simulink model "RocketSimAA"  (R2021a)
settings: Solver=VariableStepAuto  StartTime=0.0  StopTime=100  RelTol=1e-3
values from neighbouring files (symbols this model uses):
  flag_AA = 1    [main_simulation.m]
  flag_D = 1    [main_simulation.m]
  h_lim = 1000    [main_simulation.m]
  T_s = 0.01    [main_simulation.m]
undefined symbols (not defined in the file or in its folder): A_AAbig, A_AAsmall, A_R, C_DR, Controller, f_motor, g_0, H_0, h_0, h_table, m_0, m_motor, n_finAA, phi_0, R_E, rho_0, t_BO, t_data, t_motor, theta_0, v_vec
libraries: simulink x2
settings Model: SimulationMode=accelerator  Creator=SeverinBeger  LastModifiedBy=SeverinBeger

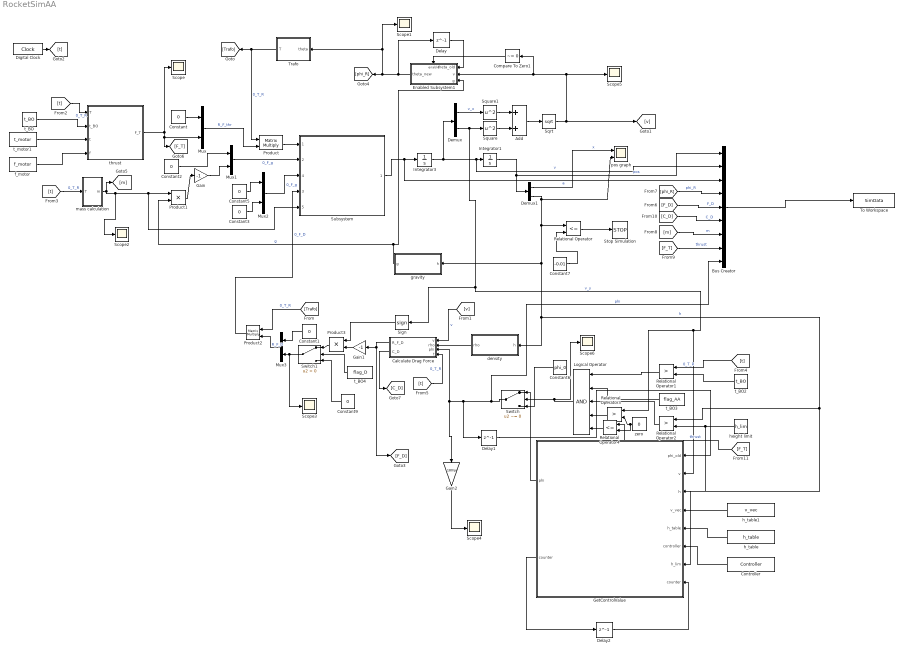
== system RocketSimAA ==
  Add : Sum
  Bus Creator : BusCreator  Inputs=9
  Calculate Drag Force : Subsystem
  Compare To Zero1 : simulink/Logic and Bit Operations/Compare To Zero  relop=~=  OutDataTypeStr=boolean
  Constant{,1..3,5,9} (6 alike) : Constant  Value=0
  Constant6 : Constant  Value=phi_0
  Constant7 : Constant  Value=-0.01
  Controller : Constant  Value=Controller
  Delay : Delay  DelayLength=1  InitialCondition=0
  Delay1 : Delay  DelayLength=1  InitialCondition=0
  Delay2 : Delay  DelayLength=1  InitialCondition=0
  Demux : Demux  Outputs=2
  Demux1 : Demux  Outputs=2
  Digital Clock : DigitalClock  SampleTime=T_s
  Enabled Subsystem1 : Subsystem  TreatAsAtomicUnit=on
  Gain : Gain  Gain=-1
  Gain1 : Gain  Gain=-1
  Gain2 : Gain  Gain=180/pi
  GetControlValue : MATLAB Function  TreatAsAtomicUnit=on
  Integrator1 : Integrator
  Integrator3 : Integrator
  Logical Operator : Logic  Inputs=5  AllPortsSameDT=off  OutDataTypeStr=boolean
  Mux{,1..3} (4 alike) : Mux  Inputs=2
  Product : Product  Multiplication=Matrix(*)
  Product1 : Product
  Product2 : Product  Multiplication=Matrix(*)
  Product3 : Product
  Relational Operator : RelationalOperator  Operator=<=  OutDataTypeStr=boolean  RndMeth=Simplest
  Relational Operator1 : RelationalOperator  Operator=>  OutDataTypeStr=boolean  RndMeth=Simplest
  Relational Operator2 : RelationalOperator  Operator=>  OutDataTypeStr=boolean  RndMeth=Simplest
  Relational Operator3 : RelationalOperator  Operator=>  OutDataTypeStr=boolean  RndMeth=Simplest
  Relational Operator4 : RelationalOperator  Operator=<=  OutDataTypeStr=boolean  RndMeth=Simplest
  Scope{,1..6} (7 alike) : Scope
  Sign : Signum
  Sqrt : Sqrt  SaturateOnIntegerOverflow=on
  Square : Math  Operator=square  SaturateOnIntegerOverflow=on
  Square1 : Math  Operator=square  SaturateOnIntegerOverflow=on
  Stop Simulation : Stop
  Subsystem : Subsystem  ReferencedSubsystem=acceleration
      settings: PortSchema="{\"entries\":[{\"content\":{\"sides\":[{\"content\":{\"connectorIds\":[\"In1\",\"In2\",\"In4\",\"In3\",\"In5\"]},\"type\":\"ConnectorPlacement.EquallySpacedRectSide\",\"uuid\":\"9ef3e48b-891b-4d0d-a708-ee121c0097dd\"},{\"content\":{\"connectorIds\":[\"Out1\"],\"side\":\"RIGHT\"},\"type\":\"ConnectorPlacement.EquallySpacedRectSide\",\"uuid\":\"fe012b3b-856e-4c20-af45-176b50db60e5\"},{\"content\":{\"connectorIds\":[],\"side\":\"TOP\"},\"type\":\"ConnectorPlacement.EquallySpacedRectSide\",\"uuid\":\"c344a42b-cb7d-481a-b552-86bd89250f10\"}]},\"type\":\"ConnectorPlacement.EquallySpacedConnector\",\"uuid\":\"b7d8efea-7233-4c8a-80e4-a1935eebb6ed\"}],\"packageUris\":[\"http://schema.mathworks.com/mf0/Connector/R2020b\"],\"version\":\"1.0\"}"
  Switch : Switch  Criteria=u2 ~= 0
  Switch1 : Switch  Criteria=u2 > Threshold
  To Workspace : ToWorkspace  VariableName=SimData  SaveFormat=Timeseries  SampleTime=-1
  Trafo : MATLAB Function  TreatAsAtomicUnit=on
  density : Subsystem
  f_motor : Constant  Value=f_motor
  gravity : Subsystem
  h_table : Constant  Value=h_table
  h_table1 : Constant  Value=v_vec
  height limit : Constant  Value=h_lim
  mass calculation : Subsystem
  pos graph : Scope  NumInputPorts=2
  t_BO : Constant  Value=t_BO
  t_BO2 : Constant  Value=t_BO
  t_BO3 : Constant  Value=flag_AA
  t_BO4 : Constant  Value=flag_D
  t_motor1 : Constant  Value=t_motor
  thrust : MATLAB Function  TreatAsAtomicUnit=on
  zero : Constant  Value=0
  wires:
  Subsystem/1 -> Bus Creator/3, Integrator3/1  "a"
  Integrator3/1 -> Demux/1, Bus Creator/2, Integrator1/1  "v"
  Integrator1/1 -> Demux1/1, Bus Creator/1  "pos"
  Demux1/2 -> Relational Operator/1, gravity/1(h), Relational Operator2/1, GetControlValue/3(h), density/1(h), pos graph/2  "h"
  Demux/2 -> Relational Operator3/1, GetControlValue/2(v), Sign/1, Square/1  "v_y"
  Demux/1 -> Square1/1  "v_x"
  thrust/1(F_T) -> [F_T], Mux/2, Scope/1
  Constant/1 -> Mux/1
  Product/1 -> Subsystem/1
  Mux/1 -> Product/2  "R_F_thr"
  Trafo/1(T) -> [Trafo], Product/1  "0_T_R"
  Constant2/1 -> Mux1/1
  Mux1/1 -> Subsystem/2  "0_F_g"
  Product1/1 -> Gain/1
  Gain/1 -> Mux1/2
  gravity/1(g) -> Enabled Subsystem1/3(g), Product1/2  "g"
  Constant5/1 -> Mux2/1
  Constant3/1 -> Mux2/2
  Mux2/1 -> Subsystem/4  "0_F_g"
  Demux1/1 -> pos graph/1  "x"
  Relational Operator/1 -> Stop Simulation/1
  Add/1 -> Sqrt/1
  Square/1 -> Add/2
  Square1/1 -> Add/1
  Sqrt/1 -> Scope5/1, Compare To Zero1/1, Enabled Subsystem1/2(v), [v]
  Delay/1 -> Enabled Subsystem1/1(theta_old)
  Compare To Zero1/1 -> Enabled Subsystem1/Enable
  Enabled Subsystem1/1(theta_new) -> Delay/1, Trafo/1(theta), Scope1/1, [phi_R]
  Constant7/1 -> Relational Operator/2
  Calculate Drag Force/1(R_F_D) -> [F_D], Gain1/1
  Constant1/1 -> Mux3/1
  Mux3/1 -> Product2/2  "R_F_D"
  [Trafo] -> Product2/1  "0_T_R"
  Product2/1 -> Subsystem/3  "0_F_D"
  [v] -> Calculate Drag Force/1(v)  "v"
  Constant6/1 -> Switch/3
  Logical Operator/1 -> Scope6/1, Switch/2
  Digital Clock/1 -> [t]
  t_BO/1 -> thrust/2(t_BO)
  [t] -> thrust/1(T)  "0_T_R"
  [t] -> Relational Operator1/1  "0_T_R"
  t_BO2/1 -> Relational Operator1/2
  Relational Operator1/1 -> Logical Operator/1
  t_BO3/1 -> Logical Operator/2
  GetControlValue/1(phi) -> Switch/1
  [t] -> Calculate Drag Force/4(t)  "0_T_R"
  Switch1/1 -> Scope3/1, Mux3/2
  t_BO4/1 -> Switch1/2
  Constant9/1 -> Switch1/3
  density/1(rho) -> Calculate Drag Force/2(rho)
  Gain1/1 -> Product3/2
  Product3/1 -> Switch1/1
  Sign/1 -> Product3/1
  Bus Creator/1 -> To Workspace/1
  [F_D] -> Bus Creator/5  "F_D"
  t_motor1/1 -> thrust/3(t)
  f_motor/1 -> thrust/4(f)
  mass calculation/1(m) -> Scope2/1, Subsystem/5, Product1/1, [m]
  [t] -> mass calculation/1(T)  "0_T_R"
  [phi_R] -> Bus Creator/4  "phi_R"
  [m] -> Bus Creator/7  "m"
  [F_T] -> Bus Creator/8  "thrust"
  Calculate Drag Force/2(C_D) -> [C_D]
  [C_D] -> Bus Creator/6  "C_D"
  Controller/1 -> GetControlValue/6(controller)
  h_table/1 -> GetControlValue/5(h_table)
  h_table1/1 -> GetControlValue/4(v_vec)
  Relational Operator2/1 -> Logical Operator/3
  Switch/1 -> Bus Creator/9, Delay1/1, Calculate Drag Force/3(phi), Gain2/1  "phi"
  height limit/1 -> GetControlValue/7(h_lim), Relational Operator2/2
  Gain2/1 -> Scope4/1
  Delay1/1 -> GetControlValue/1(phi_old)
  Relational Operator3/1 -> Logical Operator/4
  zero/1 -> Relational Operator4/2, Relational Operator3/2
  Relational Operator4/1 -> Logical Operator/5
  [F_T] -> Relational Operator4/1  "thrust"
  GetControlValue/2(counter) -> Delay2/1
  Delay2/1 -> GetControlValue/8("counter ")

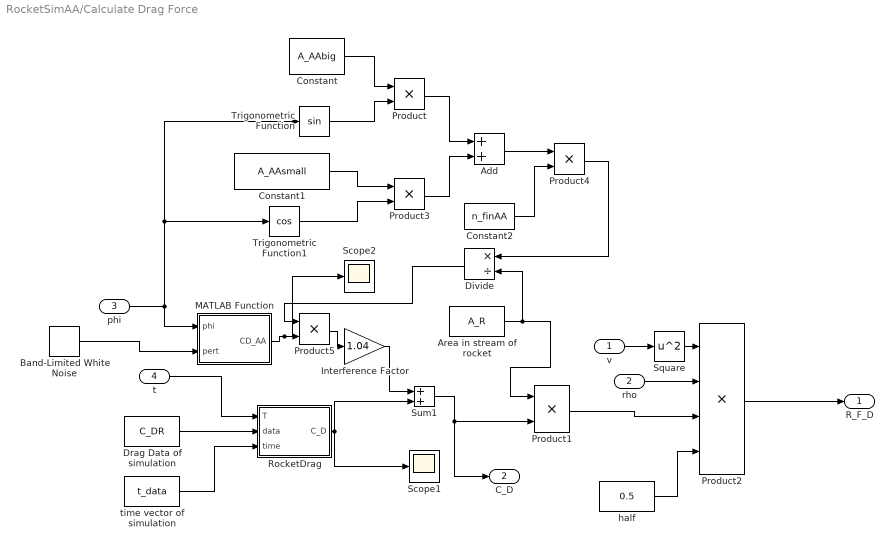
== system RocketSimAA/Calculate Drag Force ==
  v : Inport
  rho : Inport  Port=2
  phi : Inport  Port=3
  t : Inport  Port=4
  Add : Sum
  Area in stream of rocket : Constant  Value=A_R
  Band-Limited White Noise : simulink/Sources/Band-Limited White Noise  Cov=[0.1]  Ts=0.1  seed=[23341]
  Constant : Constant  Value=A_AAbig
  Constant1 : Constant  Value=A_AAsmall
  Constant2 : Constant  Value=n_finAA
  Divide : Product  Inputs=*/
  Drag Data of simulation : Constant  Value=C_DR
  Interference Factor : Gain  Gain=1.04
  MATLAB Function : MATLAB Function  TreatAsAtomicUnit=on
  Product{,1,3..5} (5 alike) : Product
  Product2 : Product  Inputs=4
  RocketDrag : MATLAB Function  TreatAsAtomicUnit=on
  Scope1 : Scope
  Scope2 : Scope
  Square : Math  Operator=square  SaturateOnIntegerOverflow=on
  Sum1 : Sum
  Trigonometric Function : Trigonometry
  Trigonometric Function1 : Trigonometry  Operator=cos
  half : Constant  Value=0.5
  time vector of simulation : Constant  Value=t_data
  R_F_D : Outport
  C_D : Outport  Port=2
  wires:
  phi/1 -> Trigonometric Function1/1, Trigonometric Function/1, MATLAB Function/1(phi)
  Area in stream of rocket/1 -> Divide/2, Product1/1
  rho/1 -> Product2/2
  Product1/1 -> Product2/3
  half/1 -> Product2/4
  Product2/1 -> R_F_D/1
  Drag Data of simulation/1 -> RocketDrag/2(data)
  time vector of simulation/1 -> RocketDrag/3(time)
  t/1 -> RocketDrag/1(T)
  RocketDrag/1(C_D) -> Sum1/2, Scope1/1
  v/1 -> Square/1
  Square/1 -> Product2/1
  Sum1/1 -> C_D/1, Product1/2
  Band-Limited White Noise/1 -> MATLAB Function/2(pert)
  Constant1/1 -> Product3/1
  Trigonometric Function1/1 -> Product3/2
  Trigonometric Function/1 -> Product/2
  Constant/1 -> Product/1
  Product3/1 -> Add/2
  Product/1 -> Add/1
  Add/1 -> Product4/1
  Constant2/1 -> Product4/2
  Product4/1 -> Divide/1
  Divide/1 -> Product5/1
  MATLAB Function/1(CD_AA) -> Scope2/1, Product5/2
  Product5/1 -> Interference Factor/1
  Interference Factor/1 -> Sum1/1

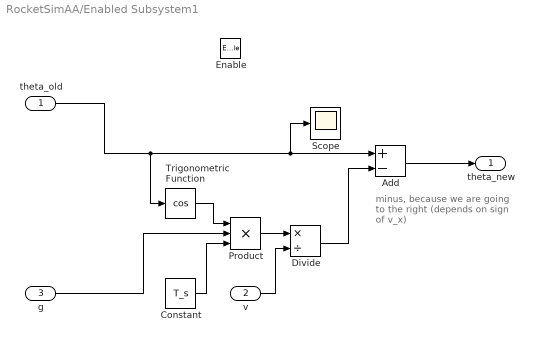
== system RocketSimAA/Enabled Subsystem1 ==
  note: minus, because we are going to the right (depends on sign of v_x)
  theta_old : Inport
  v : Inport  Port=2
  g : Inport  Port=3
  Enable : EnablePort
  Add : Sum  Inputs=+-
  Constant : Constant  Value=T_s
  Divide : Product  Inputs=*/
  Product : Product  Inputs=3
  Scope : Scope
  Trigonometric Function : Trigonometry  Operator=cos
  theta_new : Outport  InitialOutput=theta_0
  wires:
  Constant/1 -> Product/3
  Divide/1 -> Add/2
  Add/1 -> theta_new/1
  theta_old/1 -> Trigonometric Function/1, Scope/1, Add/1
  g/1 -> Product/2
  Trigonometric Function/1 -> Product/1
  v/1 -> Divide/2
  Product/1 -> Divide/1

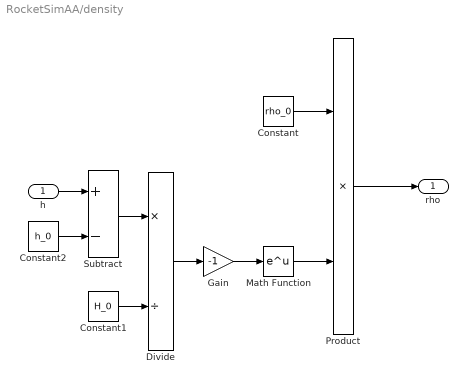
== system RocketSimAA/density ==
  h : Inport
  Constant : Constant  Value=rho_0  VectorParams1D=off
  Constant1 : Constant  Value=H_0  VectorParams1D=off
  Constant2 : Constant  Value=h_0  VectorParams1D=off
  Divide : Product  Inputs=*/
  Gain : Gain  Gain=-1
  Math Function : Math  SaturateOnIntegerOverflow=on
  Product : Product
  Subtract : Sum  Inputs=+-
  rho : Outport
  wires:
  h/1 -> Subtract/1
  Constant2/1 -> Subtract/2
  Subtract/1 -> Divide/1
  Constant1/1 -> Divide/2
  Divide/1 -> Gain/1
  Gain/1 -> Math Function/1
  Math Function/1 -> Product/2
  Constant/1 -> Product/1
  Product/1 -> rho/1

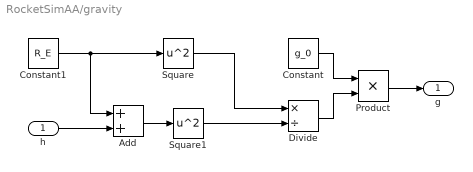
== system RocketSimAA/gravity ==
  h : Inport
  Add : Sum
  Constant : Constant  Value=g_0
  Constant1 : Constant  Value=R_E
  Divide : Product  Inputs=*/
  Product : Product
  Square : Math  Operator=square  SaturateOnIntegerOverflow=on
  Square1 : Math  Operator=square  SaturateOnIntegerOverflow=on
  g : Outport
  wires:
  h/1 -> Add/2
  Constant1/1 -> Square/1, Add/1
  Add/1 -> Square1/1
  Square/1 -> Divide/1
  Square1/1 -> Divide/2
  Divide/1 -> Product/2
  Constant/1 -> Product/1
  Product/1 -> g/1

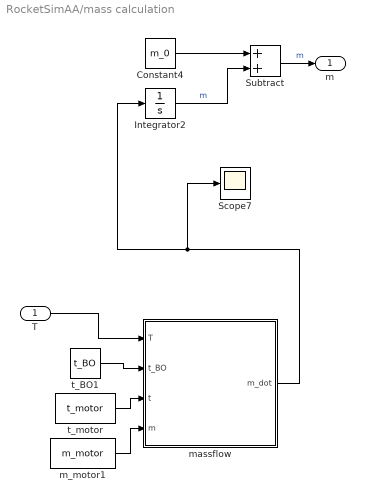
== system RocketSimAA/mass calculation ==
  T : Inport
  Constant4 : Constant  Value=m_0
  Integrator2 : Integrator
  Scope7 : Scope
  Subtract : Sum
  m_motor1 : Constant  Value=m_motor
  massflow : MATLAB Function  TreatAsAtomicUnit=on
  t_BO1 : Constant  Value=t_BO
  t_motor : Constant  Value=t_motor
  m : Outport
  wires:
  t_BO1/1 -> massflow/2(t_BO)
  massflow/1(m_dot) -> Integrator2/1, Scope7/1
  t_motor/1 -> massflow/3(t)
  Integrator2/1 -> Subtract/2  "m"
  m_motor1/1 -> massflow/4(m)
  Constant4/1 -> Subtract/1
  Subtract/1 -> m/1  "m"
  T/1 -> massflow/1(T)

== matlab function RocketSimAA/thrust ==
  data: T input; F_T output; t_BO input; t input; f input
function F_T = thrust(T,t_BO,t,f)
% this is an interpolation of the thrust for a certain rocket motor:
% O3400
%Inputs: Time T to evaluate, time of burnout of motor, t is time arre of
%motor test, f is thrust array of motor test
%Output: thrust at time T in N:  F_T(T)
F_T = 0;
    if(T <= max(t))

        % interpolate:
        t_delta = T-t;
        [min_t,idx] = min(abs(t_delta));

        if t_delta(idx) < 0
            p1 = idx-1;
            p2 = idx;
        elseif min_t > 0
            p1 = idx;
            p2 = idx + 1;
        else
            F_T = f(idx);
            return;
        end

        F_T = f(p1) + (f(p2)-f(p1))*(T-t(p1))/(t(p2)-t(p1));
    end
end

== matlab function RocketSimAA/mass calculation/massflow ==
  data: T input; m_dot output; t_BO input; t input; m input
function m_dot = massflow(T,t_BO,t,m)
% this is an interpolation of the massflow for a certain rocket motor:
% O3400
%Inputs: Time T to evaluate, time of burnout of motor, t is time array of
%motor test, m is mass array of motor test
%Output: massflow at time T in kg:  m_dot(T)
m_dot = 0;
if(T <= max(t))

    m_dot_arr = [0];

    for i=2:length(t)
        m_dot_arr = [m_dot_arr, (m(i)-m(i-1))/(t(i)-t(i-1))];
    end

    % interpolate:
    t_delta = T-t;
    [min_t,idx] = min(abs(t_delta));
    
    if t_delta(idx) < 0
        p1 = idx-1;
        p2 = idx;
    elseif min_t > 0
        p1 = idx;
        p2 = idx + 1;
    else
        m_dot = m_dot_arr(idx);
        return;
    end
    
    m_dot = m_dot_arr(p1) + (m_dot_arr(p2)-m_dot_arr(p1))*(T-t(p1))/(t(p2)-t(p1));
end
end

== matlab function RocketSimAA/Trafo ==
  data: theta input; T output
function T = Trafo(theta)
 %Transformation from the rocket coordinate system to the world system
 %(x,y)
 %Theta defines the angle between the rocket axis and the ground, defined
 %positive anticlockwise
 T = [sin(theta), cos(theta);
     -cos(theta),sin(theta)];
end

== matlab function RocketSimAA/Calculate Drag Force/MATLAB Function ==
  settings: updateMethod=DISCRETE
  data: phi input; CD_AA output; pert input
function CD_AA = fcn(phi,pert)


%inspiration:
    %https://www.researchgate.net/publication/278049906_Experimental_Investigation_on_the_Performance_of_NACA_4412_Aerofoil_with_Curved_Leading_Edge_Planform/figures?lo=1
    %https://www.grc.nasa.gov/www/k-12/rocket/shaped.html
% rng('shuffle');
%correct angle


if(phi > pi)
    disp("Angle phi of the active aero fins is wrong. Too big.");
    disp(phi*180/pi);
    CD_AA = 1.28;
    return;
elseif(-phi > pi)
    disp("Angle phi of the active aero fins is wrong. Too Small.");
    disp(phi*180/pi);
    CD_AA = 0.045;
    return;
elseif(phi>pi/2)
    phi = pi/2;
elseif(phi < 0)
    phi = 0;
end

CD_min = 0.045; %typical airfoil
CD_max = 1.28;  %typical flat plate perpendicular

phi_lim = 16; %20 degrees till stalling

if(phi *180/pi <= phi_lim)
    CD_AA = CD_min + 10*CD_min * exp(1+phi *180/pi / phi_lim)/(exp(2)); % exponential rise
    
else
    CD_base = 11*CD_min;
    CD_AA =  CD_base + ((phi*180/pi)-phi_lim)/(90-phi_lim)*(CD_max-CD_base);
    %add random perturbation
%     pert = rand(); %between 0 and 1

    CD_AA = CD_AA + sign(pert-0.5) * CD_AA./20 * pert; %randomly perturbe around 5 degrees 
    
end

== matlab function RocketSimAA/Calculate Drag Force/RocketDrag ==
  data: T input; C_D output; data input; time input
function C_D = RocketDrag(T,data,time)
% this is an interpolation of the drag coefficient of a simulation with RAS
% Aero II
%Inputs: Time T to evaluate, dragdata, time vector of the recorded data
%Output: coefficient of drag C_D
% l = length(time);
if(T>max(time))
%     C_D = mean(data(round(4/5*l):end));
    C_D = mean(data(end));
    return;
end


    % interpolate:
    t_delta = T-time;
    [min_t,idx] = min(abs(t_delta));
    
    if t_delta(idx) < 0
        p1 = idx-1;
        p2 = idx;
    elseif min_t > 0
        p1 = idx;
        p2 = idx + 1;
    else
        C_D = data(idx);
        return;
    end
    
    C_D = data(p1) + (data(p2)-data(p1))*(T-time(p1))/(time(p2)-time(p1));
end

== matlab function RocketSimAA/GetControlValue ==
  data: phi_old input; v input; phi output [0..pi/2]; h input; v_vec input; h_table input; controller input; h_lim input; counter input; counter output
function [phi,counter] = fcn(phi_old,v,h,v_vec,h_table,controller,h_lim,counter)

    phi = phi_old;
    h_idx = [];

if(h<h_lim)
    return;
end

if(v > v_vec(1)) %bigger than highest possible value -> brake as hard as possible
    phi = pi/2;
    return;
end

% [deltav,v_idx] = min((v-v_vec).^2);

% if(v_vec(v_idx) < v && v_idx ~= 0) %length(v_vec)) %%only switch phi value, if new v is bigger than v value in v_vec
%     v_idx = v_idx - 1;
% end

%% Find starting index
if(counter == 0) %find next smaller value of v
    delta_v = v-v_vec;
    delta_v_pos = delta_v > 0;
    minv = min(delta_v(delta_v_pos));
    counter_poss = find(delta_v == minv,1,'first'); % to avoid the possibility of "counter" being an array...
    counter = counter_poss(1);
end

%% Skip if over the controllers reach
if(counter >= length(v_vec)) %we are beyond the controllers reach
return;
end

%% if v is one of the discrete states -> go get a new phi
if(abs(v-v_vec(counter)) < 0.1)

    v_idx = counter;
    counter = counter+1;
    
    if(v_idx == length(v_vec)) %close to goal, keep the current angle
        return;
    end


    h_vec = h_table(v_idx,:);
        
    
    if(h < h_vec(1))
            phi = 0;
        elseif(h>h_vec(end))
            phi = pi/2;
        else
        
        % Strategy: take closest value
%         [~,h_idx] = min((h-h_vec).^2);
        %phi = controller(v_idx(1),h_idx(1)); %get new angle
        
        % Strategy: Interpolation
        [delta_h_vec,delta_h_indcs] = sort((h-h_vec).^2); %sorts it in ascending order -> 1 == lowest val
        idx1 = min(delta_h_indcs(1:2));
        idx2 = max(delta_h_indcs(1:2));
        phi1 = controller(v_idx(1),idx1(1));
        phi2 = controller(v_idx(1),idx2(1));
        phi = phi1 + (phi2-phi1)* (h-h_vec(idx1))/(h_vec(idx2)-h_vec(idx1));
        
        

        end

        %this should not happen
        if(isnan(phi)) % && ~isempty(h_idx)) %if not defined in controller -> look at distance to bounds 
    %         dist_high = abs(h_table(v_idx,h_idx) - h_table(v_idx,end));
    %         dist_low =  abs(h_table(v_idx,h_idx) - h_table(v_idx,1));
    %         if(dist_high < dist_low) %closer to upper bound -> brake
    %             phi = pi/2;
    %         else %closer to lower bound -> coast
    %             phi = 0;
    %         end
            phi = phi_old;
            return;
        end
elseif(v-v_vec(counter) < 0)
    counter = counter + 1;
    return;
end

%safety
if(phi >= pi/2)
    phi = pi/2;
elseif(phi <= 0)
    phi = 0;
end
